simulink model "top_system"  (R2022b)
settings: Solver=VariableStepAuto  StartTime=0.0  StopTime=1e-7  RelTol=1e-3
libraries: commrandsrc3 x1
settings Model: Creator=Ali-Laptop  LastModifiedBy=Ali-Laptop
settings DebuggingCC: AlgebraicLoopMsg=none

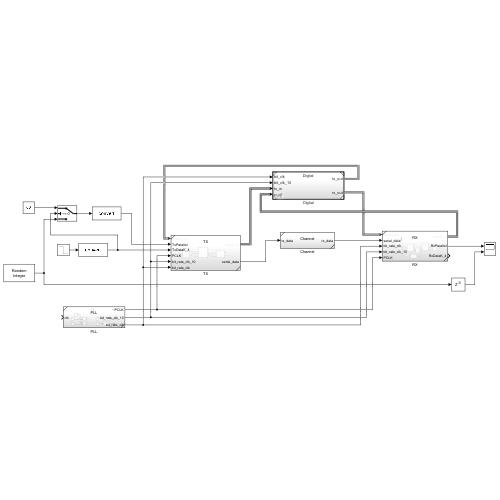
[thumbnail: Simulink's stored preview of the top-level diagram]
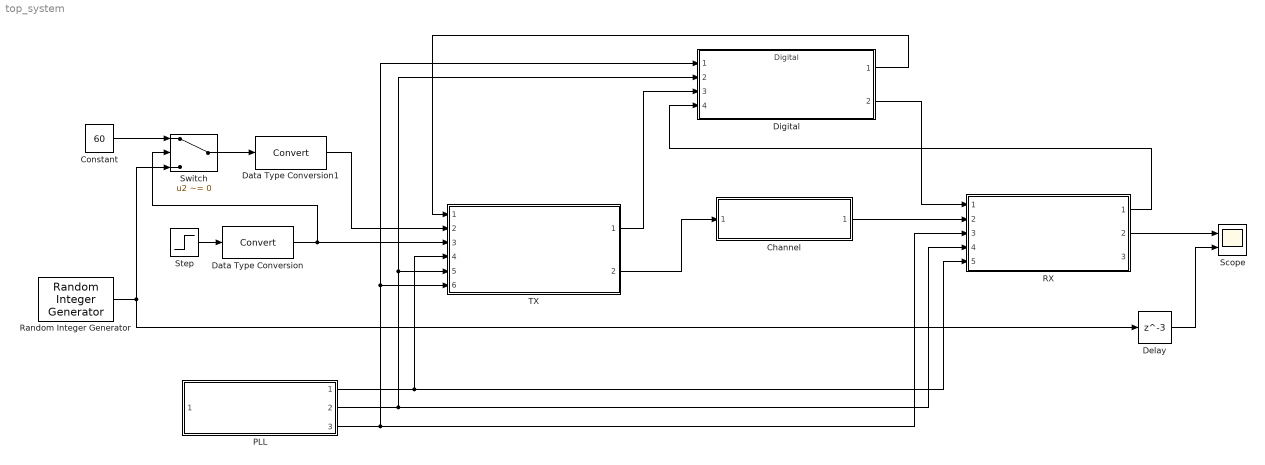
== system top_system ==
  Channel : Subsystem  ReferencedSubsystem=Channel
  Constant : Constant  Value=60  SampleTime=2e-9
  Data Type Conversion : DataTypeConversion  SaturateOnIntegerOverflow=off  RndMeth=Floor
  Data Type Conversion1 : DataTypeConversion  SaturateOnIntegerOverflow=off  RndMeth=Floor
  Delay : Delay  DelayLength=3
  Digital : ModelReference  ModelNameDialog=Digital.slx  SimulationMode=Normal  ModelReferenceVersion=1.6
  PLL : Subsystem  ReferencedSubsystem=PLL
  RX : Subsystem  ReferencedSubsystem=RX
  Random Integer Generator : commrandsrc3/Random Integer Generator  SetSize=256  SeedSource=Auto  Seed=0  SampleTime=2e-9  SamplesPerFrame=1  OutputDataType=uint8  SimulateUsing=Interpreted execution
  Scope : Scope  NumInputPorts=2
  Step : Step  Time=2e-9  Before=1  After=0  OutDataTypeStr=Inherit: Inherit via back propagation  SampleTime=1e-10
  Switch : Switch  Criteria=u2 ~= 0  SaturateOnIntegerOverflow=off  InputSameDT=off
  TX : Subsystem  ReferencedSubsystem=TX
  wires:
  PLL/1 -> RX/5, TX/4
  PLL/2 -> RX/4, Digital/2, TX/5
  PLL/3 -> RX/3, Digital/1, TX/6
  Digital/2 -> RX/1
  RX/1 -> Digital/4
  Channel/1 -> RX/2
  TX/2 -> Channel/1
  Step/1 -> Data Type Conversion/1
  RX/2 -> Scope/1
  Digital/1 -> TX/1
  TX/1 -> Digital/3
  Data Type Conversion/1 -> TX/3, Switch/2
  Switch/1 -> Data Type Conversion1/1
  Random Integer Generator/1 -> Delay/1, Switch/3
  Constant/1 -> Switch/1
  Data Type Conversion1/1 -> TX/2
  Delay/1 -> Scope/2
